simulink model "learn"  (R2022b)
settings: Solver=VariableStepAuto  StartTime=0.0  StopTime=500  RelTol=1e-3  AbsTol=1e-3
undefined symbols (not defined in the file): duct_W, T_set, tube_D
libraries: fl_lib x41, nesl_utility x15, SimscapeFluids_lib x8, simulink_extras x2
(part 2 of 2)

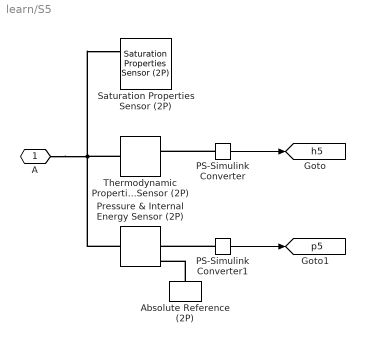
== system learn/S5 ==
  Absolute Reference (2P) : fl_lib/Two-Phase Fluid/Elements/Absolute Reference (2P)
  PS-Simulink Converter : nesl_utility/PS-Simulink Converter  PhysicalDomain=network_engine_domain  SubClassName=ps_output  LeftPortType=input  RightPortType=output  PseudoPeriodic=off  Frequencies=[]  VectorFormat=inherit  Unit=kJ/kg  AffineConversion=off
  PS-Simulink Converter1 : nesl_utility/PS-Simulink Converter  PhysicalDomain=network_engine_domain  SubClassName=ps_output  LeftPortType=input  RightPortType=output  PseudoPeriodic=off  Frequencies=[]  VectorFormat=inherit  Unit=MPa  AffineConversion=off
  Pressure & Internal Energy Sensor (2P) : fl_lib/Two-Phase Fluid/Sensors/Pressure & Internal Energy Sensor (2P)
      settings: InternalSimscapePortConfiguration="{\"Bottom\":[],\"Left\":[{\"id\":\"A\",\"label\":\"A\",\"type\":\"foundation.two_phase_fluid.two_phase_fluid\"}],\"Right\":[{\"id\":\"B\",\"label\":\"B\",\"type\":\"foundation.two_phase_fluid.two_phase_fluid\"},{\"id\":\"P\",\"label\":\"P\",\"type\":\"output\"},{\"id\":\"U\",\"label\":\"U\",\"type\":\"output\"}],\"Top\":[]}"
  Saturation Properties Sensor (2P) : fl_lib/Two-Phase Fluid/Sensors/Saturation Properties Sensor (2P)  pressure_measure=simscape.enum.onoff.off  pressure_check=simscape.enum.assert.action.error  energy_measure=foundation.enum.EnergyMeasurement.SaturatedEnthalpy  density_measure=foundation.enum.DensityMeasurement.Off
      settings: InternalSimscapePortConfiguration="{\"Bottom\":[],\"Left\":[{\"id\":\"A\",\"label\":\"A\",\"type\":\"foundation.two_phase_fluid.two_phase_fluid\"}],\"Right\":[{\"id\":\"T_sat_liq\",\"label\":\"TL\",\"type\":\"output\"},{\"id\":\"T_sat_vap\",\"label\":\"TV\",\"type\":\"output\"}],\"Top\":[{\"id\":\"h_sat_liq\",\"label\":\"HL\",\"type\":\"output\"},{\"id\":\"h_sat_vap\",\"label\":\"HV\",\"type\":\"output\"}]}"
  Thermodynamic Properties Sensor (2P) : fl_lib/Two-Phase Fluid/Sensors/Thermodynamic Properties Sensor (2P)
      settings: InternalSimscapePortConfiguration="{\"Bottom\":[],\"Left\":[{\"id\":\"A\",\"label\":\"A\",\"type\":\"foundation.two_phase_fluid.two_phase_fluid\"}],\"Right\":[{\"id\":\"T\",\"label\":\"T\",\"type\":\"output\"},{\"id\":\"H\",\"label\":\"h\",\"type\":\"output\"},{\"id\":\"V\",\"label\":\"v\",\"type\":\"output\"},{\"id\":\"S\",\"label\":\"s\",\"type\":\"output\"}],\"Top\":[]}"
  A : PMIOPort  Side=Left
  tag scope: h5=global, p5=global
  wires:
  PS-Simulink Converter/1 -> [h5]
  PS-Simulink Converter1/1 -> [p5]
  connections:
  Pressure & Internal Energy Sensor (2P)/LConn1 -- Saturation Properties Sensor (2P)/LConn1 -- Thermodynamic Properties Sensor (2P)/LConn1 -- A/RConn1
  Absolute Reference (2P)/LConn1 -- Pressure & Internal Energy Sensor (2P)/RConn1
  PS-Simulink Converter/LConn1 -- Thermodynamic Properties Sensor (2P)/RConn2
  PS-Simulink Converter1/LConn1 -- Pressure & Internal Energy Sensor (2P)/RConn2

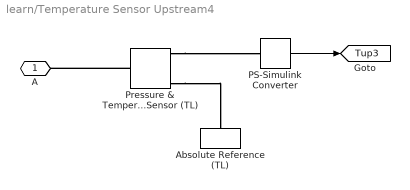
== system learn/Temperature Sensor Upstream4 ==
  Absolute Reference (TL) : fl_lib/Thermal Liquid/Elements/Absolute Reference (TL)
  PS-Simulink Converter : nesl_utility/PS-Simulink Converter  PhysicalDomain=network_engine_domain  SubClassName=ps_output  LeftPortType=input  RightPortType=output  PseudoPeriodic=off  Frequencies=[]  VectorFormat=1-D array  Unit=1  AffineConversion=off
  Pressure & Temperature Sensor (TL) : fl_lib/Thermal Liquid/Sensors/Pressure & Temperature Sensor (TL)
      settings: InternalSimscapePortConfiguration="{\"Bottom\":[],\"Left\":[{\"id\":\"A\",\"label\":\"A\",\"type\":\"foundation.thermal_liquid.thermal_liquid\"}],\"Right\":[{\"id\":\"B\",\"label\":\"B\",\"type\":\"foundation.thermal_liquid.thermal_liquid\"},{\"id\":\"P\",\"label\":\"P\",\"type\":\"output\"},{\"id\":\"T\",\"label\":\"T\",\"type\":\"output\"}],\"Top\":[]}"
  A : PMIOPort  Side=Left
  tag scope: Tup3=global
  wires:
  PS-Simulink Converter/1 -> [Tup3]
  connections:
  Pressure & Temperature Sensor (TL)/LConn1 -- A/RConn1
  Pressure & Temperature Sensor (TL)/RConn3 -- PS-Simulink Converter/LConn1
  Pressure & Temperature Sensor (TL)/RConn1 -- Absolute Reference (TL)/LConn1

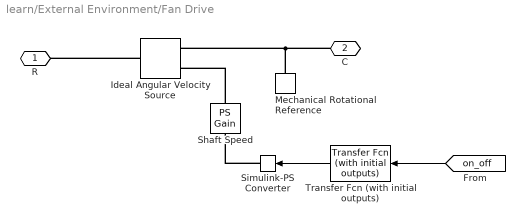
== system learn/External Environment/Fan Drive ==
  Ideal Angular Velocity Source : fl_lib/Mechanical/Mechanical Sources/Ideal Angular Velocity Source
  Mechanical Rotational Reference : fl_lib/Mechanical/Rotational Elements/Mechanical Rotational Reference
  Shaft Speed : fl_lib/Physical Signals/Functions/PS Gain  gain=3000 rpm
  Simulink-PS Converter : nesl_utility/Simulink-PS Converter  PhysicalDomain=network_engine_domain  SubClassName=ps_input  LeftPortType=input  RightPortType=output  PseudoPeriodic=off  Frequencies=[]  NoiseDistribution=none  NoiseParameters=[]  Unit=1  AffineConversion=off  FilteringAndDerivatives=provide  SimscapeFilterOrder=1  InputFilterTimeConstant=0.001  UdotUserProvided=0
  Transfer Fcn (with initial outputs) : simulink_extras/Additional Linear/Transfer Fcn (with initial outputs)  N=[1]  D="[2  1]"  Y0=1  U0=0
  R : PMIOPort  Side=Left
  C : PMIOPort  Port=2  Side=Right
  wires:
  Transfer Fcn (with initial outputs)/1 -> Simulink-PS Converter/1
  [on_off] -> Transfer Fcn (with initial outputs)/1
  connections:
  Ideal Angular Velocity Source/LConn1 -- R/RConn1
  Shaft Speed/RConn1 -- Ideal Angular Velocity Source/RConn1
  Simulink-PS Converter/RConn1 -- Shaft Speed/LConn1
  C/RConn1 -- Mechanical Rotational Reference/LConn1 -- Ideal Angular Velocity Source/RConn2
